simulink model "krazekPrzykladSimulink"  (R2018a)
settings: Solver=VariableStepAuto  StartTime=0.0  StopTime=1  RelTol=1e-3
settings Model: Creator=Mateusz  LastModifiedBy=Mateusz

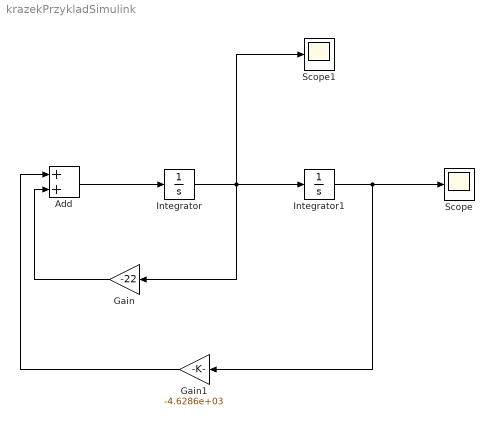
== system krazekPrzykladSimulink ==
  Add : Sum
  Gain : Gain  Gain=-22
  Gain1 : Gain  Gain=-4.6286e+03
  Integrator : Integrator
  Integrator1 : Integrator  InitialCondition=0.1
  Scope : Scope
  Scope1 : Scope
  wires:
  Integrator1/1 -> Gain1/1, Scope/1
  Add/1 -> Integrator/1
  Gain/1 -> Add/2
  Integrator/1 -> Scope1/1, Gain/1, Integrator1/1
  Gain1/1 -> Add/1
